simulink model "Target_Vehicle_Speed"  (R2022b)
settings: configuration reference "CommonModelConfiguration" (kept outside this file)
undefined symbols (not defined in the file): cc_param_160, cc_param_23
settings Model: Creator=rkallum  LastModifiedBy=OTHOMSO1
settings ConfigSetRef: SourceName=CommonModelConfiguration  SourceLocation=Base Workspace

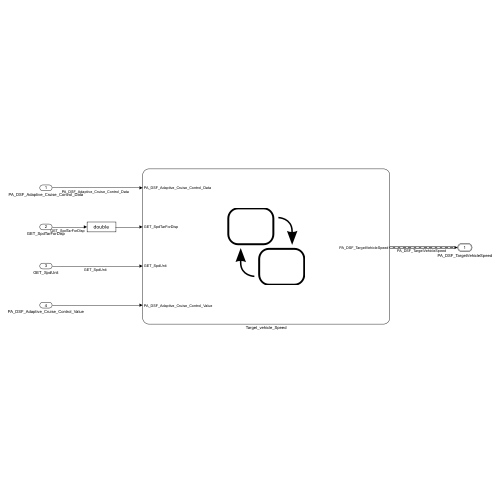
[thumbnail: Simulink's stored preview of the top-level diagram]
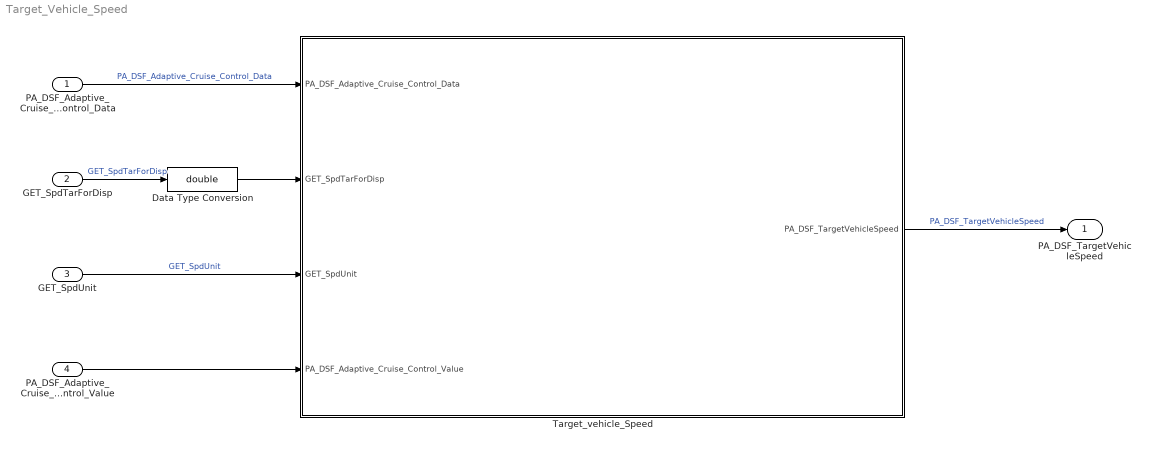
== system Target_Vehicle_Speed ==
  PA_DSF_Adaptive_Cruise_Control_Data : Inport  OutDataTypeStr=Enum: E_DSF_Data
  GET_SpdTarForDisp : Inport  Port=2  OutDataTypeStr=Spd31
  GET_SpdUnit : Inport  Port=3  OutDataTypeStr=Enum: VehSpdIndcdUnit
  PA_DSF_Adaptive_Cruise_Control_Value : Inport  Port=4  OutDataTypeStr=Enum: E_DSF_Value
  Data Type Conversion : DataTypeConversion  OutDataTypeStr=double  SaturateOnIntegerOverflow=off  RndMeth=Floor
  Target_vehicle_Speed : Stateflow chart  TreatAsAtomicUnit=on
  PA_DSF_TargetVehicleSpeed : Outport  OutDataTypeStr=Bus: StatusAndIntValue  VectorParamsAs1DForOutWhenUnconnected=off
  wires:
  PA_DSF_Adaptive_Cruise_Control_Data/1 -> Target_vehicle_Speed/1(PA_DSF_Adaptive_Cruise_Control_Data)  "PA_DSF_Adaptive_Cruise_Control_Data"
  GET_SpdTarForDisp/1 -> Data Type Conversion/1  "GET_SpdTarForDisp"
  GET_SpdUnit/1 -> Target_vehicle_Speed/3(GET_SpdUnit)  "GET_SpdUnit"
  Target_vehicle_Speed/1(PA_DSF_TargetVehicleSpeed) -> PA_DSF_TargetVehicleSpeed/1  "PA_DSF_TargetVehicleSpeed"
  Data Type Conversion/1 -> Target_vehicle_Speed/2(GET_SpdTarForDisp)
  PA_DSF_Adaptive_Cruise_Control_Value/1 -> Target_vehicle_Speed/4(PA_DSF_Adaptive_Cruise_Control_Value)

== stateflow chart Target_Vehicle_Speed/Target_vehicle_Speed ==
  state CARCONFIG_INVALID
    entry: PA_DSF_TargetVehicleSpeed.Status=E_CommonStatus.NotPresent
    PA_DSF_TargetVehicleSpeed.Value=int32(0);
  state SYSTEM_OK
    state NOT_ACTIVE
      entry: PA_DSF_TargetVehicleSpeed.Status=E_CommonStatus.Disabled
      PA_DSF_TargetVehicleSpeed.Value=int32(0);
    state ACTIVE
      entry: PA_DSF_TargetVehicleSpeed.Status=E_CommonStatus.Available
      state retval=getConvertToHmiSpeed(SpeedInMs) [function]
        state retval1=convertFromMs(speedinms) [function]
          (default) -> (junction 135)
          (junction 135) -> (junction 136) [order 1] : [GET_SpdUnit==VehSpdIndcdUnit.VehSpdIndcdUnit_Kmph]
          (junction 135) -> (junction 137) [order 2] : {retval1=speedinms*1152/515}
          (junction 136) -> (junction 138) : {retval1=speedinms*36/10}
          (junction 138) -> (junction 137)
          (junction 137) -> (junction 139)
        state ConvertedSpeed = getConvertedSpeed(ConfigMid, ConfigTop, Speed, BreakpointMid, BreakpointTop) [function]
          (default) -> (junction 153)
          (junction 153) -> (junction 154) [order 1] : [Speed==0]
          (junction 153) -> (junction 155) [order 2]
          (junction 154) -> (junction 159) : {ConvertedSpeed=0}
          (junction 155) -> (junction 156) [order 1] : [Speed<=BreakpointMid]
          (junction 155) -> (junction 157) [order 2] : {ConvertedSpeed=Speed+(Speed-BreakpointMid)*(ConfigTop-ConfigMid)/(BreakpointTop-BreakpointMid)+ConfigMid}
          (junction 156) -> (junction 158) : {ConvertedSpeed=Speed+(Speed*ConfigMid/BreakpointMid)}
          (junction 158) -> (junction 157)
          (junction 159) -> (junction 158)
          (junction 157) -> (junction 160)
        (default) -> (junction 115)
        (junction 115) -> (junction 114) [order 1] : [cc_param_160==1 || cc_param_160==3 || cc_param_160==5]
        (junction 114) -> (junction 120) : {retval=convertFromMs(SpeedInMs)}
        (junction 115) -> (junction 116) [order 2]
        (junction 116) -> (junction 117) [order 1] : [GET_SpdUnit==VehSpdIndcdUnit.VehSpdIndcdUnit_Kmph]
        (junction 116) -> (junction 118) [order 2] : {retval=getConvertedSpeed(1.12, 3.6,convertFromMs(SpeedInMs), 24.86, 161.56)}
        (junction 117) -> (junction 119) : {retval=getConvertedSpeed(1.8, 5.8,convertFromMs(SpeedInMs), 40, 260)}
        (junction 119) -> (junction 118)
        (junction 120) -> (junction 119)
        (junction 118) -> (junction 121)
      (default) -> (junction 177)
      ACTIVE -> (junction 177) [order 1]
      (junction 177) -> (junction 175) [order 1] : [GET_SpdUnit==VehSpdIndcdUnit.VehSpdIndcdUnit_Kmph]
      (junction 175) -> (junction 180) [order 1] : [getConvertToHmiSpeed(GET_SpdTarForDisp) >= 260]
          | {PA_DSF_TargetVehicleSpeed.Value = int32(260);}
      (junction 177) -> (junction 186) [order 2]
      (junction 175) -> (junction 176) [order 2]
      (junction 180) -> (junction 188)
      (junction 186) -> (junction 176) [order 2]
      (junction 176) -> (junction 188) : {PA_DSF_TargetVehicleSpeed.Value=int32(getConvertToHmiSpeed(GET_SpdTarForDisp));}
      (junction 186) -> (junction 178) [order 1] : [getConvertToHmiSpeed(GET_SpdTarForDisp) >= 160]
          | {PA_DSF_TargetVehicleSpeed.Value = int32(160);}
      (junction 188) -> (junction 190)
      (junction 178) -> (junction 190)
      (junction 190) -> (junction 172)
    (default) -> NOT_ACTIVE
    NOT_ACTIVE -> ACTIVE : [(PA_DSF_Adaptive_Cruise_Control_Data~=E_DSF_Data.DSF_CruiseOverridden &&...
        | PA_DSF_Adaptive_Cruise_Control_Data~=E_DSF_Data.DSF_NoTarget) &&...
        | PA_DSF_Adaptive_Cruise_Control_Value==E_DSF_Value.DSF_Active]
    ACTIVE -> NOT_ACTIVE [order 1] : [(PA_DSF_Adaptive_Cruise_Control_Data==E_DSF_Data.DSF_CruiseOverridden ||...
        | PA_DSF_Adaptive_Cruise_Control_Data==E_DSF_Data.DSF_NoTarget) ||...
        | PA_DSF_Adaptive_Cruise_Control_Value~=E_DSF_Value.DSF_Active]
  (default) -> (junction 6)
  (junction 6) -> CARCONFIG_INVALID [order 2]
  (junction 6) -> SYSTEM_OK [order 1] : [cc_param_23> 2]
  data: speedinms function_input; retval1 function_output; ConfigMid function_input; ConfigTop function_input; Speed function_input; ConvertedSpeed function_output; BreakpointMid function_input; BreakpointTop function_input; SpeedInMs function_input; retval function_output; PA_DSF_Adaptive_Cruise_Control_Data input Enum: E_DSF_Data; GET_SpdTarForDisp input double; GET_SpdUnit input Enum: VehSpdIndcdUnit; PA_DSF_TargetVehicleSpeed output Bus: StatusAndIntValue =0; cc_param_23 parameter; cc_param_160 parameter; PA_DSF_Adaptive_Cruise_Control_Value input Enum: E_DSF_Value
